simulink model "simulacion"  (R2023a)
settings: Solver=VariableStepAuto  StartTime=0.0  StopTime=10.0  RelTol=1e-3
values from neighbouring files (symbols this model uses):
  C = C0 + Cb + speed*C1    [get_matrixes.m]
  force_mask_x = zeros(number_of_nodes*4, 1)    [DEFINE.m]
  force_mask_y = zeros(number_of_nodes*4, 1)    [DEFINE.m]
  K = K0 + Kb + speed*K1    [get_matrixes.m]
  Ki = 4*k_*Ib/g^2*(1+cos(alpha))    [DEFINE.m]
  Ky = 4*k_*Ib^2/g^3*(1+cos(alpha))    [DEFINE.m]
  M = M0 + Mb    [get_matrixes.m]
settings Model: Creator=viori  LastModifiedBy=Violeta Rivera

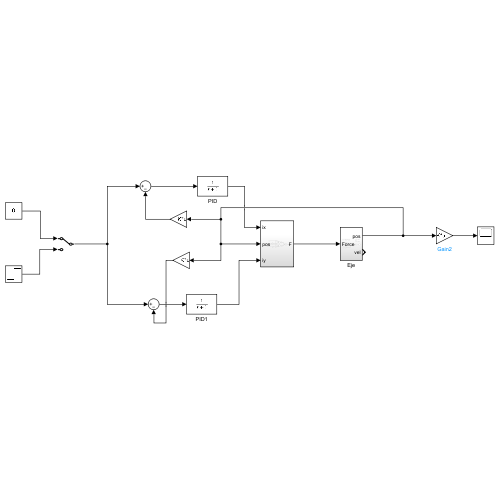
[thumbnail: Simulink's stored preview of the top-level diagram]
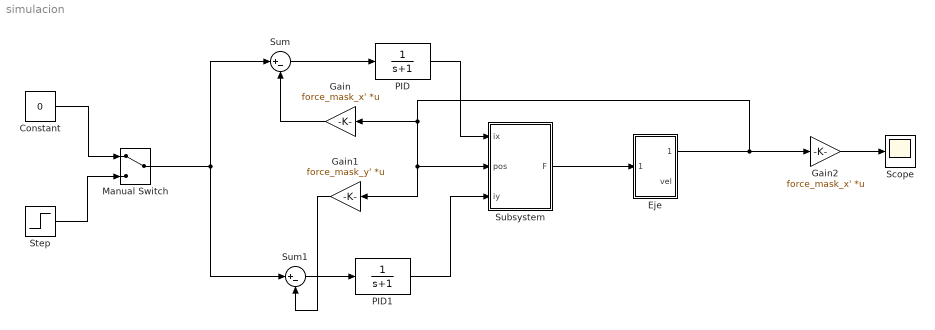
== system simulacion ==
  Constant : Constant  Value=0
  Eje : Subsystem
  Gain : Gain  Gain=force_mask_x'  Multiplication=Matrix(K*u)
  Gain1 : Gain  Gain=force_mask_y'  Multiplication=Matrix(K*u)
  Gain2 : Gain  Gain=force_mask_x'  Multiplication=Matrix(K*u)
  Manual Switch : ManualSwitch
  PID : TransferFcn  Denominator=[1 1]
  PID1 : TransferFcn  Denominator=[1 1]
  Scope : Scope
  Step : Step  SampleTime=0
  Subsystem : Subsystem
  Sum : Sum  Inputs=|+-
  Sum1 : Sum  Inputs=|+-
  wires:
  Sum/1 -> PID/1
  Subsystem/1(F) -> Eje/1(Force)
  Eje/1(pos) -> Gain2/1, Gain1/1, Subsystem/2(pos), Gain/1
  PID/1 -> Subsystem/1(ix)
  PID1/1 -> Subsystem/3(iy)
  Sum1/1 -> PID1/1
  Gain/1 -> Sum/2
  Gain1/1 -> Sum1/2
  Gain2/1 -> Scope/1
  Manual Switch/1 -> Sum1/1, Sum/1
  Constant/1 -> Manual Switch/1
  Step/1 -> Manual Switch/2

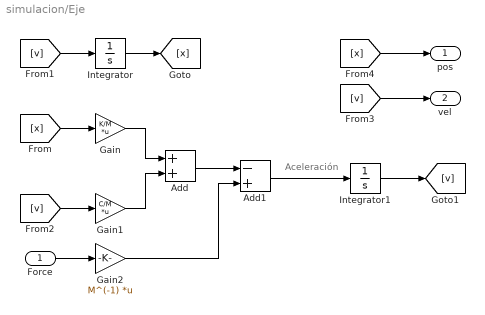
== system simulacion/Eje ==
  note: Aceleración
  Force : Inport
  Add : Sum
  Add1 : Sum  Inputs=-+
  Gain : Gain  Gain=K/M  Multiplication=Matrix(K*u)
  Gain1 : Gain  Gain=C/M  Multiplication=Matrix(K*u)
  Gain2 : Gain  Gain=M^(-1)  Multiplication=Matrix(K*u) (u vector)
  Integrator : Integrator
  Integrator1 : Integrator
  pos : Outport
  vel : Outport  Port=2
  wires:
  [x] -> Gain/1
  [v] -> Gain1/1
  Integrator/1 -> [x]
  Gain/1 -> Add/1
  Gain1/1 -> Add/2
  [v] -> Integrator/1
  Integrator1/1 -> [v]
  Add/1 -> Add1/1
  Add1/1 -> Integrator1/1
  Force/1 -> Gain2/1
  Gain2/1 -> Add1/2
  [v] -> vel/1
  [x] -> pos/1

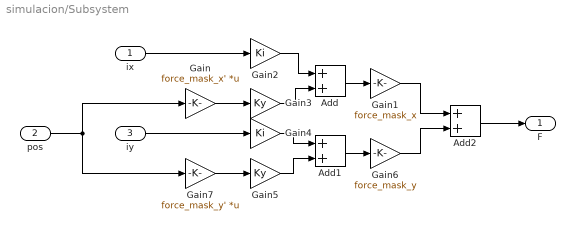
== system simulacion/Subsystem ==
  ix : Inport
  pos : Inport  Port=2
  iy : Inport  Port=3
  Add : Sum
  Add1 : Sum
  Add2 : Sum
  Gain : Gain  Gain=force_mask_x'  Multiplication=Matrix(K*u)
  Gain1 : Gain  Gain=force_mask_x
  Gain2 : Gain  Gain=Ki
  Gain3 : Gain  Gain=Ky
  Gain4 : Gain  Gain=Ki
  Gain5 : Gain  Gain=Ky
  Gain6 : Gain  Gain=force_mask_y
  Gain7 : Gain  Gain=force_mask_y'  Multiplication=Matrix(K*u)
  F : Outport
  wires:
  ix/1 -> Gain2/1
  Gain7/1 -> Gain5/1
  Gain4/1 -> Add1/1
  Gain/1 -> Gain3/1
  Gain3/1 -> Add/2
  Gain2/1 -> Add/1
  iy/1 -> Gain4/1
  Gain5/1 -> Add1/2
  Add/1 -> Gain1/1
  Add1/1 -> Gain6/1
  Gain1/1 -> Add2/1
  Gain6/1 -> Add2/2
  Add2/1 -> F/1
  pos/1 -> Gain7/1, Gain/1
